simulink model "sway_linear"  (R2020a)
settings: Solver=VariableStepAuto  StartTime=0.0  StopTime=500  RelTol=1e-3
settings Model: Creator=xiaoran  LastModifiedBy=xiaoran

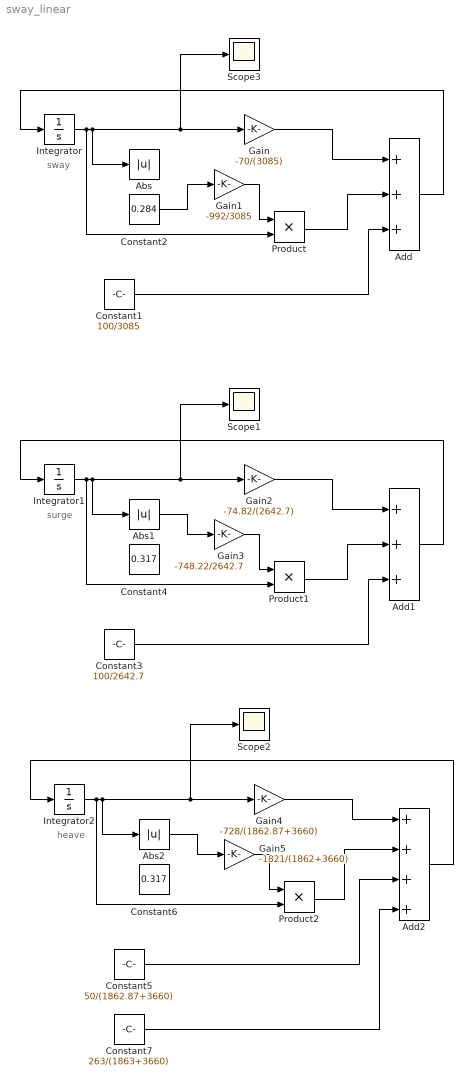
== system sway_linear ==
  note: sway
  note: surge
  note: heave
  Abs : Abs
  Abs1 : Abs
  Abs2 : Abs
  Add : Sum  Inputs=+++
  Add1 : Sum  Inputs=+++
  Add2 : Sum  Inputs=++++
  Constant1 : Constant  Value=100/3085
  Constant2 : Constant  Value=0.284
  Constant3 : Constant  Value=100/2642.7
  Constant4 : Constant  Value=0.317
  Constant5 : Constant  Value=50/(1862.87+3660)
  Constant6 : Constant  Value=0.317
  Constant7 : Constant  Value=263/(1863+3660)
  Gain : Gain  Gain=-70/(3085)
  Gain1 : Gain  Gain=-992/3085
  Gain2 : Gain  Gain=-74.82/(2642.7)
  Gain3 : Gain  Gain=-748.22/2642.7
  Gain4 : Gain  Gain=-728/(1862.87+3660)
  Gain5 : Gain  Gain=-1821/(1862+3660)
  Integrator : Integrator  InitialCondition=.1
  Integrator1 : Integrator  InitialCondition=.1
  Integrator2 : Integrator  InitialCondition=.1
  Product : Product
  Product1 : Product
  Product2 : Product
  Scope1 : Scope
  Scope2 : Scope
  Scope3 : Scope
  wires:
  Integrator/1 -> Product/2, Abs/1, Scope3/1, Gain/1
  Gain1/1 -> Product/1
  Gain/1 -> Add/1
  Product/1 -> Add/2
  Constant1/1 -> Add/3
  Add/1 -> Integrator/1
  Constant2/1 -> Gain1/1
  Add1/1 -> Integrator1/1
  Constant3/1 -> Add1/3
  Product1/1 -> Add1/2
  Gain2/1 -> Add1/1
  Gain3/1 -> Product1/1
  Integrator1/1 -> Gain2/1, Scope1/1, Abs1/1, Product1/2
  Abs1/1 -> Gain3/1
  Abs2/1 -> Gain5/1
  Integrator2/1 -> Product2/2, Abs2/1, Scope2/1, Gain4/1
  Gain5/1 -> Product2/1
  Gain4/1 -> Add2/1
  Product2/1 -> Add2/2
  Constant5/1 -> Add2/3
  Add2/1 -> Integrator2/1
  Constant7/1 -> Add2/4
